simulink model "simulretard"  (R2021b)
settings: Solver=VariableStepAuto  StartTime=0.0  StopTime=10  RelTol=1e-3
libraries: simulink x2
settings Model: Creator=alexa  LastModifiedBy=alexa

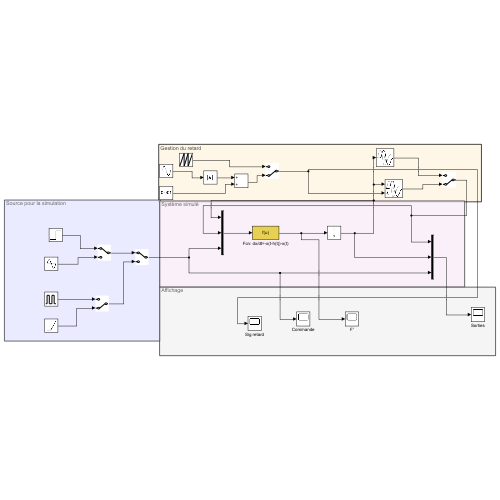
[thumbnail: Simulink's stored preview of the top-level diagram]
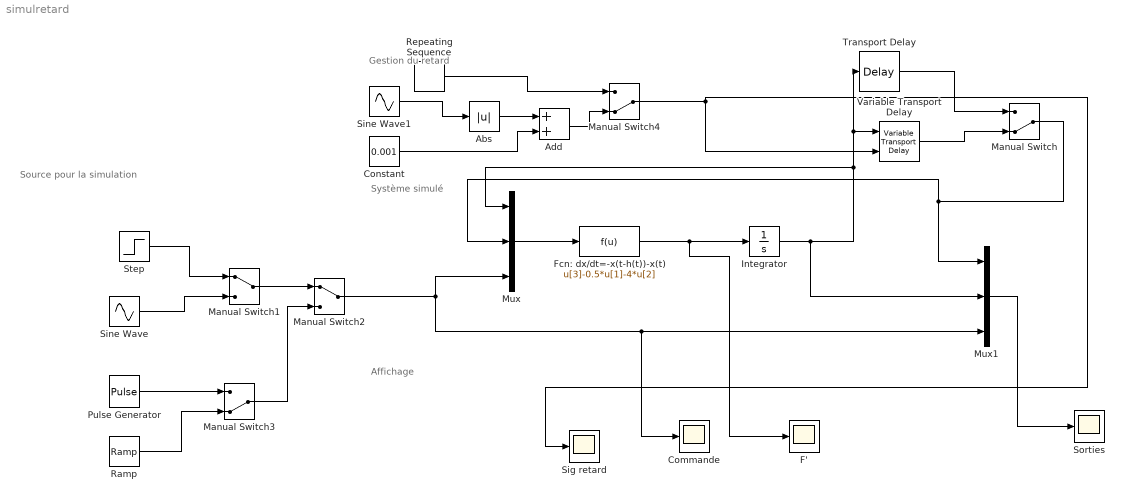
== system simulretard ==
  note: Affichage
  note: Système simulé
  note: Gestion du retard
  note: Source pour la simulation
  Abs : Abs
  Add : Sum
  Commande : Scope
  Constant : Constant  Value=0.001
  F' : Scope
  Fcn: dx/dt=-x(t-h(t))-x(t) : Fcn  Expr=u[3]-0.5*u[1]-4*u[2]
  Integrator : Integrator
  Manual Switch : ManualSwitch  CurrentSetting=0
  Manual Switch1 : ManualSwitch
  Manual Switch2 : ManualSwitch
  Manual Switch3 : ManualSwitch  CurrentSetting=0
  Manual Switch4 : ManualSwitch  CurrentSetting=0
  Mux : Mux  Inputs=3
  Mux1 : Mux  Inputs=3
  Pulse Generator : DiscretePulseGenerator  PulseType=Time based  Amplitude=10  Period=10  PulseWidth=75  PhaseDelay=1
  Ramp : simulink/Sources/Ramp  slope=1  start=0  InitialOutput=0
  Repeating Sequence : simulink/Sources/Repeating Sequence  rep_seq_t=[0 5]  rep_seq_y=[0.1 10]
  Sig retard : Scope
  Sine Wave : Sin  Amplitude=10  SampleTime=0
  Sine Wave1 : Sin  SineType=Sample based  Amplitude=2  Frequency=0.3*2*pi  Samples=100  SampleTime=0.01  Offset=1
  Sorties : Scope
      settings: Tag=Scope retard
  Step : Step  After=10  SampleTime=0
  Transport Delay : TransportDelay  DelayTime=5
  Variable Transport Delay : VariableTransportDelay  VariableDelayType=Variable transport delay  MaximumDelay=15
  wires:
  Mux/1 -> Fcn: dx/dt=-x(t-h(t))-x(t)/1
  Fcn: dx/dt=-x(t-h(t))-x(t)/1 -> F'/1, Integrator/1
  Integrator/1 -> Mux1/2, Transport Delay/1, Variable Transport Delay/1, Mux/1
  Mux1/1 -> Sorties/1
  Transport Delay/1 -> Manual Switch/1
  Variable Transport Delay/1 -> Manual Switch/2
  Manual Switch/1 -> Mux1/1, Mux/2
  Step/1 -> Manual Switch1/1
  Sine Wave/1 -> Manual Switch1/2
  Manual Switch1/1 -> Manual Switch2/1
  Manual Switch2/1 -> Mux/3, Commande/1, Mux1/3
  Pulse Generator/1 -> Manual Switch3/1
  Ramp/1 -> Manual Switch3/2
  Manual Switch3/1 -> Manual Switch2/2
  Repeating Sequence/1 -> Manual Switch4/1
  Manual Switch4/1 -> Sig retard/1, Variable Transport Delay/2
  Sine Wave1/1 -> Abs/1
  Constant/1 -> Add/2
  Abs/1 -> Add/1
  Add/1 -> Manual Switch4/2
